simulink model "IFFT_Stream_Ex1"  (R2024a)
settings: Solver=VariableStepAuto  StartTime=0.0  StopTime=0.1  RelTol=1e-3
undefined symbols (not defined in the file): None, S, vsva2197, xcvc1902
libraries: dspxfrm3 x2, aieUtilities x2, aieDSP x1, dspsrcs4 x1, vmcUtilities x1
settings Model: Creator=sdegala  LastModifiedBy=robg
settings ModelReferenceCC: EnableRefExpFcnMdlSchedulingChecks=on
settings RTWCC: GPUComputeCapability=3.5
settings ConfigComp: CovBoundaryAbsTol=1.0e-5

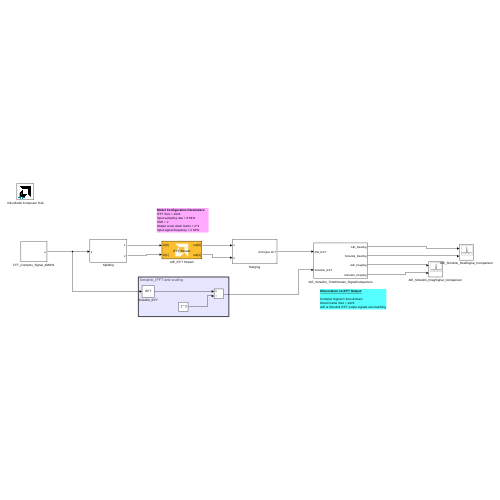
[thumbnail: Simulink's stored preview of the top-level diagram]
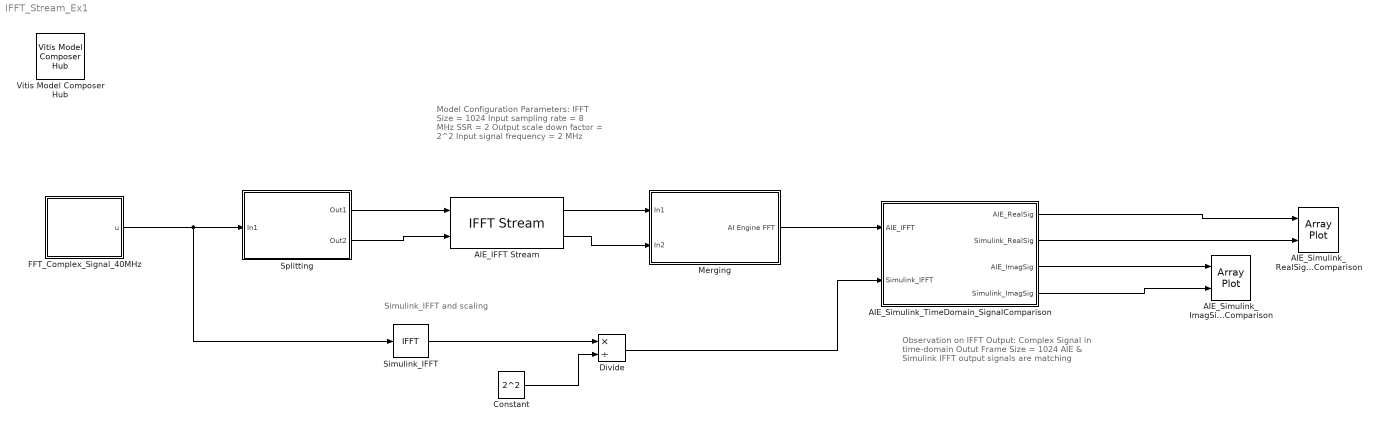
== system IFFT_Stream_Ex1 ==
  note: Model Configuration Parameters:
      | IFFT Size = 1024
      | Input sampling rate = 8 MHz
      | SSR = 2
      | Output scale down factor = 2^2
      | Input signal frequency = 2 MHz
  note: Simulink_IFFT and scaling
  note: Observation on IFFT Output:
      |
      | Complex Signal in time-domain
      | Outut Frame Size = 1024
      | AIE & Simulink IFFT output signals are matching
  AIE_IFFT Stream : aieDSP/IFFT Stream  data_type=cint16  data_out_type=cint16  twiddle_type=cint16  point_size=1024  input_window_size=1024  shift_val=2  rnd_mode=Round symmetrical to infinity  sat_mode=0-None  ssr=2  twiddle_mode=0  use_ssr_widget_kernels=off  casc_length=1  AIE_VARIANT=1  transform_fft_nifft=0  TP_API=1  TP_DYN_PT_SIZE=0  blockJsonConstraints=[]  blockJsonConstraintsInternal=[]  spec=vmc_stream_ifft.json  SerializedMaskParamNames=[]  SerializedMaskParamValues=[]  SerializedMaskParamVisibilities=[]  block_type=IFFT Stream  SerializedMaskParamDataypes=typename|typename|typename|uint|uint|uint|uint|uint|uint|uint|uint|uint|uint|uint|uint|uint  SerializedMaskParamEnumStrArr=0|0|0|0|0|0|Round to positive infinity,Round to negative infinity,Round symmetrical to infinity,Round symmetrical to zero,Round convergent to even,Round convergent to odd|0-None,1-Asymmetric,3-Symmetric|0|0|0|0|0|0|0|0  SerializedMaskParamEnumValArr=0|0|0|0|0|0|2,3,4,5,6,7|0,1,3|0|0|0|0|0|0|0|0  SerializedMaskParamVectorArr=0|0|0|0|0|0|0|0|0|0|0|0|0|0|0|0  SerializedMaskParamKeys=TT_DATA|TT_OUT_DATA|TT_TWIDDLE|TP_POINT_SIZE|TP_WINDOW_VSIZE|TP_SHIFT|TP_RND|TP_SAT|TP_PARALLEL_POWER|TP_TWIDDLE_MODE|TP_USE_WIDGETS|TP_CASC_LEN|AIE_VARIANT|TP_FFT_NIFFT|TP_API|TP_DYN_PT_SIZE
  "AIE_Simulink_ImagSignal_Comparison " : ArrayPlot  NumInputPorts=2  WindowPosition=[2.000000,37.000000,1280.000000,655.000000,]  PlotType=Line  YLimits=[-1280,1280]  ShowLegend=on
  AIE_Simulink_RealSignal_Comparison : ArrayPlot  NumInputPorts=2  WindowPosition=[2.000000,37.000000,1280.000000,655.000000,]  PlotType=Line  YLimits=[-1281.125,1280.125]  ShowLegend=on
  AIE_Simulink_TimeDomain_SignalComparison : Subsystem
  Constant : Constant  Value=2^2  OutDataTypeStr=int16
  Divide : Product  Inputs=*/  OutDataTypeStr=int16
  FFT_Complex_Signal_40MHz : Subsystem
  Merging : Subsystem
  Simulink_IFFT : dspxfrm3/IFFT  FFTImplementation=Auto  CompMethod=Table lookup  TableOpt=NEW  TableOptActive=Speed  BitRevOrder=off  cs_in=off  Normalize=off  InheritFFTLength=off  FFTLength=1024  WrapInput=on  mode=Complex  outSamplingMode=Sample based  roundingMode=Floor  overflowMode=off  firstCoeffDataTypeStr=Inherit: Same word length as input  firstCoeffLastDataTypeStr=Inherit: Same word length as input  prodOutputMode=Binary point scaling  prodOutputWordLength=32  prodOutputFracLength=0  prodOutputDataTypeStr=fixdt(1,32,0)  prodOutputLastDataTypeStr=fixdt(1,32,0)  outputMode=Binary point scaling  outputWordLength=32  outputFracLength=0  outputDataTypeStr=fixdt(1,32,0)  outputMin=[]  outputMax=[]  outputLastDataTypeStr=fixdt(1,32,0)
  Splitting : Subsystem
  Vitis Model Composer Hub : vmcUtilities/Vitis Model Composer Hub  Tag=genX  CodeGeneration=off  StartColumn=1  NumberOfColumns=1  TargetDirectory=./code  exportDesign=off  analyzeDesign=off  validateDesignOnHw=off  ExportType=AI Engines  IpVendor=xilinx.com  IpLibrary=hls  IpVersion=1.0  IpHWLanguage=Verilog  AieCompilerOptions={}  AieSimulatorOptions={}  CreateTestbench=off  TestbenchStackSize=10  RunRtlSim=off  RunCSim=off  RunAieSim=off  AieSimTimeout=50000  RunAieSimProfiling=off  LaunchVitisAnalyzer=off  PlotOutput=off  RunX86Sim=off  X86SimTimeout=10  GenHwImage=off  GenLibadfXo=off  GenHwValidationCode=off  PlatformType=Not Specified  HwSystemType=Baremetal  HwValidationTarget=hw  ProjDevice=xcvc1902-vsva2197-1LP-e-S  ProjDevicePart=xcvc1902-vsva2197-1LP-e-S  AIEType=AIE  SamplePeriod=-1  ClockFrequency=200  DataPathParallelism=1  xilinxfamily=versalaicore  part=xcvc1902  speed=-1LP-e-S  package=vsva2197  directory=./netlist  testbench=off  incr_netlist=off  synthesis_tool=Vivado  clock_wrapper=Clock Enables  dbl_ovrd=According to Block Masks  dcm_input_clock_period=10  sysclk_period=10  simulink_period=1  eval_field=0  LogFileName=''  NThreads=4
  wires:
  AIE_Simulink_TimeDomain_SignalComparison/3(AIE_ImagSig) -> "AIE_Simulink_ImagSignal_Comparison "/1
  AIE_Simulink_TimeDomain_SignalComparison/1(AIE_RealSig) -> AIE_Simulink_RealSignal_Comparison/1
  AIE_Simulink_TimeDomain_SignalComparison/2(Simulink_RealSig) -> AIE_Simulink_RealSignal_Comparison/2
  AIE_Simulink_TimeDomain_SignalComparison/4(Simulink_ImagSig) -> "AIE_Simulink_ImagSignal_Comparison "/2
  Splitting/1(Out1) -> AIE_IFFT Stream/1
  Splitting/2(Out2) -> AIE_IFFT Stream/2
  AIE_IFFT Stream/1 -> Merging/1(In1)
  AIE_IFFT Stream/2 -> Merging/2(In2)
  Merging/1(AI Engine FFT) -> AIE_Simulink_TimeDomain_SignalComparison/1(AIE_IFFT)
  Divide/1 -> AIE_Simulink_TimeDomain_SignalComparison/2(Simulink_IFFT)
  FFT_Complex_Signal_40MHz/1(u) -> Simulink_IFFT/1, Splitting/1(In1)
  Constant/1 -> Divide/2
  Simulink_IFFT/1 -> Divide/1

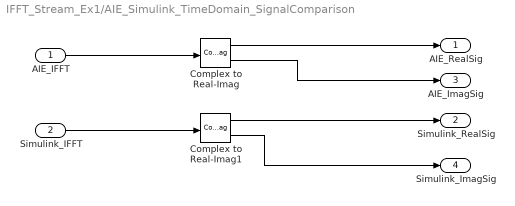
== system IFFT_Stream_Ex1/AIE_Simulink_TimeDomain_SignalComparison ==
  AIE_IFFT : Inport
  Simulink_IFFT : Inport  Port=2
  Complex to Real-Imag : ComplexToRealImag
  Complex to Real-Imag1 : ComplexToRealImag
  AIE_RealSig : Outport
  Simulink_RealSig : Outport  Port=2
  AIE_ImagSig : Outport  Port=3
  Simulink_ImagSig : Outport  Port=4
  wires:
  AIE_IFFT/1 -> Complex to Real-Imag/1
  Complex to Real-Imag/1 -> AIE_RealSig/1
  Complex to Real-Imag1/1 -> Simulink_RealSig/1
  Complex to Real-Imag1/2 -> Simulink_ImagSig/1
  Complex to Real-Imag/2 -> AIE_ImagSig/1
  Simulink_IFFT/1 -> Complex to Real-Imag1/1

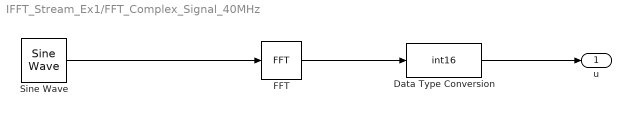
== system IFFT_Stream_Ex1/FFT_Complex_Signal_40MHz ==
  Data Type Conversion : DataTypeConversion  OutDataTypeStr=int16  ConvertRealWorld=Stored Integer (SI)  SaturateOnIntegerOverflow=off  RndMeth=Floor
  FFT : dspxfrm3/FFT  FFTImplementation=Auto  CompMethod=Table lookup  TableOpt=NEW  TableOptActive=Speed  BitRevOrder=off  Normalize=off  InheritFFTLength=on  FFTLength=64  WrapInput=on  roundingMode=Floor  overflowMode=off  firstCoeffDataTypeStr=Inherit: Same word length as input  firstCoeffLastDataTypeStr=Inherit: Same word length as input  outputMin=[]  outputMax=[]
  Sine Wave : dspsrcs4/Sine Wave  Amplitude=4  Frequency=2e6  Phase=0  SampleMode=Discrete  OutComplex=Complex  CompMethod=Trigonometric fcn  TableSize=Speed  SampleTime=1/8e6  SamplesPerFrame=1024  ResetState=Restart at time zero  OutputFrames=off  dataType=single  wordLen=16  udDataType=sfix(16)  fracBitsMode=Best precision  numFracBits=15  OutDataTypeStr=single  LastOutDataTypeStr=single
  u : Outport
  wires:
  Sine Wave/1 -> FFT/1
  FFT/1 -> Data Type Conversion/1
  Data Type Conversion/1 -> u/1

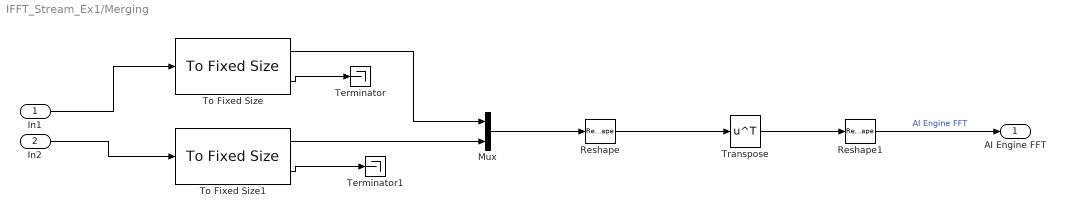
== system IFFT_Stream_Ex1/Merging ==
  In1 : Inport
  In2 : Inport  Port=2
  Mux : Mux  Inputs=2
  Reshape : Reshape  OutputDimensionality=Customize  OutputDimensions=[512, 2]
  Reshape1 : Reshape  OutputDimensions=[1, 10]
  Terminator : Terminator
  Terminator1 : Terminator
  To Fixed Size : aieUtilities/To Fixed Size  Mode=Produce a valid output signal  OutputSize=Inherit: Same as input  CopyMethod=Buffer samples to form output  HasStatusOutput=on
  To Fixed Size1 : aieUtilities/To Fixed Size  Mode=Produce a valid output signal  OutputSize=Inherit: Same as input  CopyMethod=Buffer samples to form output  HasStatusOutput=on
  Transpose : Math  Operator=transpose
  AI Engine FFT : Outport
  wires:
  Reshape/1 -> Transpose/1
  To Fixed Size1/2 -> Terminator1/1
  To Fixed Size1/1 -> Mux/2
  In2/1 -> To Fixed Size1/1
  To Fixed Size/2 -> Terminator/1
  Transpose/1 -> Reshape1/1
  To Fixed Size/1 -> Mux/1
  Mux/1 -> Reshape/1
  Reshape1/1 -> AI Engine FFT/1  "AI Engine FFT"
  In1/1 -> To Fixed Size/1

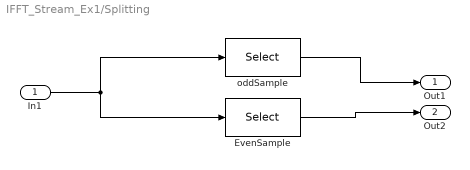
== system IFFT_Stream_Ex1/Splitting ==
  In1 : Inport
  EvenSample : Selector  InputPortWidth=1024  IndexOptions=Index vector (dialog)  Indices=2:2:1024  OutputSizes=1
  oddSample : Selector  InputPortWidth=1024  IndexOptions=Index vector (dialog)  Indices=1:2:1024  OutputSizes=1
  Out1 : Outport
  Out2 : Outport  Port=2
  wires:
  In1/1 -> oddSample/1, EvenSample/1
  EvenSample/1 -> Out2/1
  oddSample/1 -> Out1/1
